simulink model "rtwdemo_importstruct"  (Simulink 7.6)
settings: Solver=FixedStepDiscrete  StartTime=0.0  StopTime=48  FixedStep=0.01  RelTol=1e-3
PostLoadFcn:
  | %Load data into workspace
  | rtwdemo_importstruct_data;
values from neighbouring files (symbols this model uses):
  GAIN = ECoderDemos.Parameter    [rtwdemo_importstruct_data.m]
  OFFSET = ECoderDemos.Parameter    [rtwdemo_importstruct_data.m]
libraries: rtwdemowidgets x3
Description:
  | Import Externally Defined Parameters Into Simulink(R)
  | 
  | This model demonstrates how to generate code that accesses the fields of a data structure.
  | The data structure is defined in legacy (hand-written) code and accessed via pointer.
  | 
  | This technique enables users to easily switch between complete sets of parameters at run-time
  | (e.g., reference & working versions).
settings Model: Creator=The MathWorks Inc.  CovMetricSettings=d  ExtModeTrigMode=oneshot  ExtModeArmWhenConnect=off  ExtModeAutoUpdateStatusClock=off
settings MATStruct: SampleTime=0.01  Offset=0  Priority=[20.0]
settings DataIOCC: LimitDataPoints=off  SaveOutput=off  SignalLogging=off  SaveTime=off  SignalLoggingName=sigsOut
settings OptimizationCC: InlineParams=on  InlineInvariantSignals=on  PassReuseOutputArgsAs=Individual arguments  StateBitsets=on  DataBitsets=on  UseTempVars=on  ZeroExternalMemoryAtStartup=off  ZeroInternalMemoryAtStartup=off  NoFixptDivByZeroProtection=on  EfficientFloat2IntCast=on  EfficientMapNaN2IntZero=off  OptimizeModelRefInitCode=on  LifeSpan=1
settings DebuggingCC: SolverPrmCheckMsg=none  IntegerOverflowMsg=none  StrictBusMsg=ErrorOnBusTreatedAsVector
settings HardwareCC: ProdIntDivRoundTo=Zero  ProdEndianess=LittleEndian  ProdHWDeviceType=Generic->32-bit Embedded Processor  TargetHWDeviceType=Generic->32-bit Embedded Processor
settings RTWCC: SystemTargetFile=ert.tlc  TLCOptions=-aWarnNonSaturatedBlocks=0 -p0  TemplateMakefile=ert_default_tmf  Description=Real-Time Workshop Embedded Coder (no auto configuration)  GenerateReport=on  RTWVerbose=off  ProcessScript=ert_make_rtw_hook  CustomSource=rtwdemo_importstruct_user.c  IncludeHyperlinkInReport=on  LaunchReport=on
settings RTWCC: CustomInitializer=|
  | /* Initialize the volatile memory data set before switching to it */
  | Init_WorkingStruct();
settings CodeAppCC: ForceParamTrailComments=on  IgnoreCustomStorageClasses=off  IgnoreTestpoints=on  SimulinkDataObjDesc=on  CustomSymbolStrGlobalVar=rt$N$M  CustomSymbolStrType=$N$M  CustomSymbolStrFcn=$N$M$F  CustomSymbolStrMacro=$N$M  InsertBlockDesc=on
settings ERTTargetCC: TargetFcnLib=ansi_tfl_tmw.mat  MultiwordLength=2048  GenerateSampleERTMain=on  IncludeMdlTerminateFcn=off  SupportNonFinite=off  SupportComplex=off  InlinedParameterPlacement=NonHierarchical  ERTCustomFileTemplate=example_file_process.tlc  ConvertIfToSwitch=off

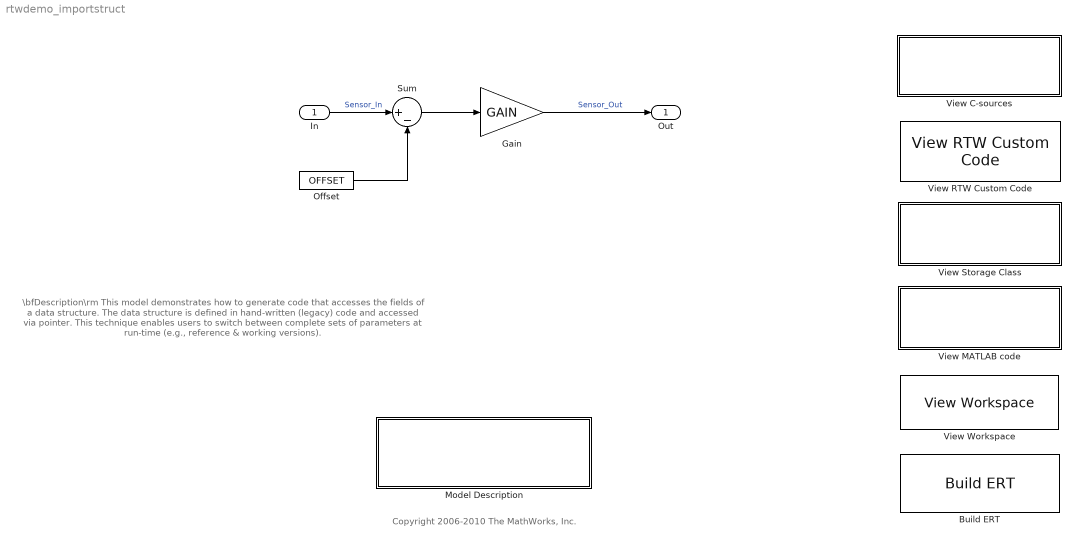
== system rtwdemo_importstruct ==
  note: \bfDescription\rm
      | This model demonstrates how to generate code that accesses the fields of a data structure.
      | The data structure is defined in hand-written (legacy) code and accessed via pointer.
      |
      | This technique enables users to switch between complete sets of parameters at run-time
      | (e.g., reference & working versions).
  note: Copyright 2006-2010 The MathWorks, Inc.
  In : Inport  OutDataTypeStr=int16  PortDimensions=[1,1]  SampleTime=0.01  Interpolate=off
  Build ERT : rtwdemowidgets/Build ERT  SystemSampleTime=-1  attrib_overrides={}
  Gain : Gain  Gain=GAIN  SampleTime=0.01  OutDataTypeStr=Inherit: Same as input  ParamDataTypeStr=Inherit: Same as input
  Model Description : Subsystem
      mask Display: disp(['Model\nDescription\n (double-click)'])
  Offset : Constant  Value=OFFSET  VectorParams1D=off
  Sum : Sum  Inputs=|+-  SampleTime=0.01  OutDataTypeStr=Inherit: Same as first input
  View C-sources : Subsystem
      settings: OpenFcn=|
      | edit rtwdemo_importstruct_user.h
      | edit rtwdemo_importstruct_user.c
      mask Display: disp(['View User C-files \n Containing Imported Struct \n(double-click)']);
  View MATLAB code : Subsystem
      settings: OpenFcn=edit rtwdemo_importstruct_data.m
      mask Display: disp(['View MATLAB program For\nCreating Variables\n(double-click)']);
  View RTW Custom Code : rtwdemowidgets/View RTW Custom Code  SystemSampleTime=-1
  View Storage Class : Subsystem  Description=cscdesigner
      settings: OpenFcn=cscdesigner ECoderDemos
      mask Type: Custom storage class designer
      mask Description: Custom storage class designer for defining custom storage classes and memory sections inside a package.
      mask Help: helpview([docroot,'/toolbox/ecoder/helptargets.map'],'data_obj_wiz');
      mask Display: disp('Custom Storage Class\nDefinition\n(double-click)');
  View Workspace : rtwdemowidgets/View Workspace  SystemSampleTime=-1
  Out : Outport  OutDataTypeStr=int16  PortDimensions=[1,1]
  wires:
  Sum/1 -> Gain/1
  Gain/1 -> Out/1  "Sensor_Out"
  In/1 -> Sum/1  "Sensor_In"
  Offset/1 -> Sum/2

== system rtwdemo_importstruct/Model Description ==
  note: \bfInstructions\rm
      |
      | 1. Inspect the handwritten user C-files containing the struct by double-clicking "View User C-files" in the model.
      |     Look at the header file "rtwdemo\_importstruct\_user.h" and the source file "rtwdemo\_importstruct\_user.c".
      |
      | 2. Look at the "Custom Code Configuration" by double-clicking the corresponding button in the model.
      |     Inspect the "Initialize function" of the "Include custom c-code in generated" section to see how to add
      |     custom initialization function calls to the generated code. To see how to include custom C-files, look at
      |     "Source files" in the "Include list of additional" section.
      |
      | 3. View the custom storage class of the ECoderDemos package used in the model  by double-clicking
      |      "Custom Storage Class Definition" in the model, and then selecting "StructPointer". Inspect the settings
      |      of the tabs "General" and "Structure Attributes". Change the attributes and watch the changes in the
      |      preview window. Note that you can specify the pointer name within the data object itself by setting the
      |      struct name to "Instance specific".
      |
      | 4. Open the MATLAB program used to generate the data objects by double-clicking "View MATLAB code for Generating
      |     Variables" in the model. This file is executed by referencing it in the PostLoadFcn Callback of the
      |     "Model properties" dialog.
      |
      | 5. Look at the workspace variables by clicking the "View Workspace Variables" button to the right.
      |
      | 6. Generate code for this example by double-clicking "Generate Code" in the model. The code
      |      generation report will appear. Open the model C-file "rtwdemo\_importstruct.c". Inspect the model step
      |      function "rtwdemo\_importstruct\_step". Notice the user-specific code in the model initialize function
      |     "rtwdemo\_importstruct\_initialize".

== system rtwdemo_importstruct/View C-sources ==

== system rtwdemo_importstruct/View MATLAB code ==

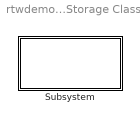
== system rtwdemo_importstruct/View Storage Class ==
  Subsystem : Subsystem

== system rtwdemo_importstruct/View Storage Class/Subsystem ==
